simulink library "EMD"  (R2021b)
settings: Solver=VariableStepAuto  StartTime=0.0  StopTime=10.0  RelTol=1e-3
libraries: $bdroot x2
settings Model: Creator=Szalay  LastModifiedBy=Szalay

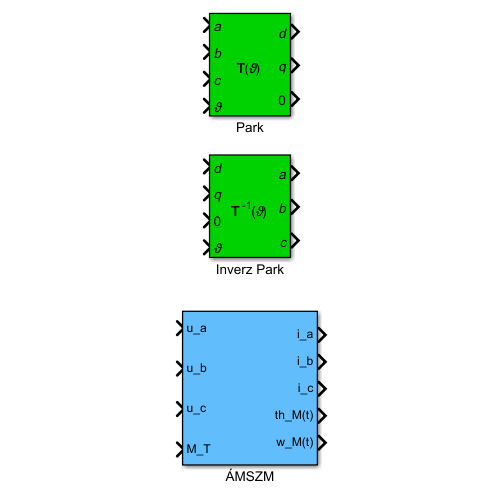
[thumbnail: Simulink's stored preview of the top-level diagram]
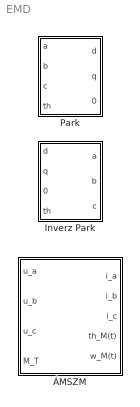
== system EMD ==
  Inverz Park : Subsystem
      mask Display:
      | % Bemenetek
      | port_label('input', 1, '\itd', 'texmode', 'on');
      | port_label('input', 2, '\itq', 'texmode', 'on');
      | port_label('input', 3, '0', 'texmode', 'on');
      | 
      | port_label('input', 4, '\it\vartheta', 'texmode', 'on');
      | 
      | % Kimenetek
      | port_label('output', 1, '\ita', 'texmode', 'on');
      | port_label('output', 2, '\itb', 'texmode', 'on');
      | port_label('output', 3, '\itc', 'texmode', 'on');
      | 
      | % Felirat
      | text( ...
      | 	0.5, 0.5, '{\bfT}^{ -1}({\it\vartheta})', ...
      | 	'texmode', 'on', ...
      | 	'HorizontalAlignment', 'center' ...
      | 	);
  Park : Subsystem
      mask Display:
      | % Bemenetek
      | port_label('input', 1, '\ita', 'texmode', 'on');
      | port_label('input', 2, '\itb', 'texmode', 'on');
      | port_label('input', 3, '\itc', 'texmode', 'on');
      | 
      | port_label('input', 4, '\it\vartheta', 'texmode', 'on');
      | 
      | % Kimenetek
      | port_label('output', 1, '\itd', 'texmode', 'on');
      | port_label('output', 2, '\itq', 'texmode', 'on');
      | port_label('output', 3, '0', 'texmode', 'on');
      | 
      | % Felirat
      | text( ...
      | 	0.5, 0.5, '{\bfT}({\it\vartheta})', ...
      | 	'texmode', 'on', ...
      | 	'HorizontalAlignment', 'center' ...
      | 	);
  ÁMSZM : Subsystem

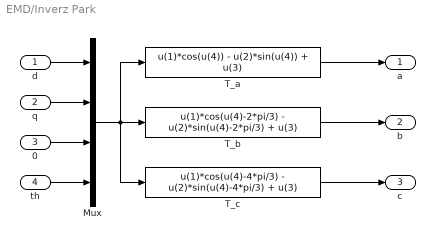
== system EMD/Inverz Park ==
  d : Inport
  q : Inport  Port=2
  0 : Inport  Port=3
  th : Inport  Port=4
  Mux : Mux
  T_a : MATLABFcn  MATLABFcn=u(1)*cos(u(4)) - u(2)*sin(u(4)) + u(3)
  T_b : MATLABFcn  MATLABFcn=u(1)*cos(u(4)-2*pi/3) - u(2)*sin(u(4)-2*pi/3) + u(3)
  T_c : MATLABFcn  MATLABFcn=u(1)*cos(u(4)-4*pi/3) - u(2)*sin(u(4)-4*pi/3) + u(3)
  a : Outport
  b : Outport  Port=2
  c : Outport  Port=3
  wires:
  0/1 -> Mux/3
  d/1 -> Mux/1
  th/1 -> Mux/4
  T_c/1 -> c/1
  q/1 -> Mux/2
  T_b/1 -> b/1
  T_a/1 -> a/1
  Mux/1 -> T_b/1, T_c/1, T_a/1

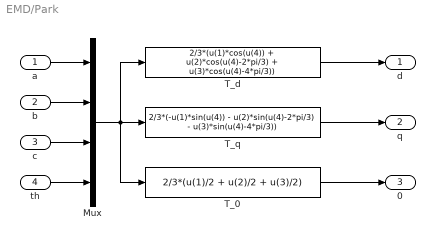
== system EMD/Park ==
  a : Inport
  b : Inport  Port=2
  c : Inport  Port=3
  th : Inport  Port=4
  Mux : Mux
  T_0 : MATLABFcn  MATLABFcn=2/3*(u(1)/2 + u(2)/2 + u(3)/2)
  T_d : MATLABFcn  MATLABFcn=2/3*(u(1)*cos(u(4)) + u(2)*cos(u(4)-2*pi/3) + u(3)*cos(u(4)-4*pi/3))
  T_q : MATLABFcn  MATLABFcn=2/3*(-u(1)*sin(u(4)) - u(2)*sin(u(4)-2*pi/3) - u(3)*sin(u(4)-4*pi/3))
  d : Outport
  q : Outport  Port=2
  0 : Outport  Port=3
  wires:
  Mux/1 -> T_d/1, T_0/1, T_q/1
  T_d/1 -> d/1
  T_q/1 -> q/1
  b/1 -> Mux/2
  T_0/1 -> 0/1
  th/1 -> Mux/4
  a/1 -> Mux/1
  c/1 -> Mux/3

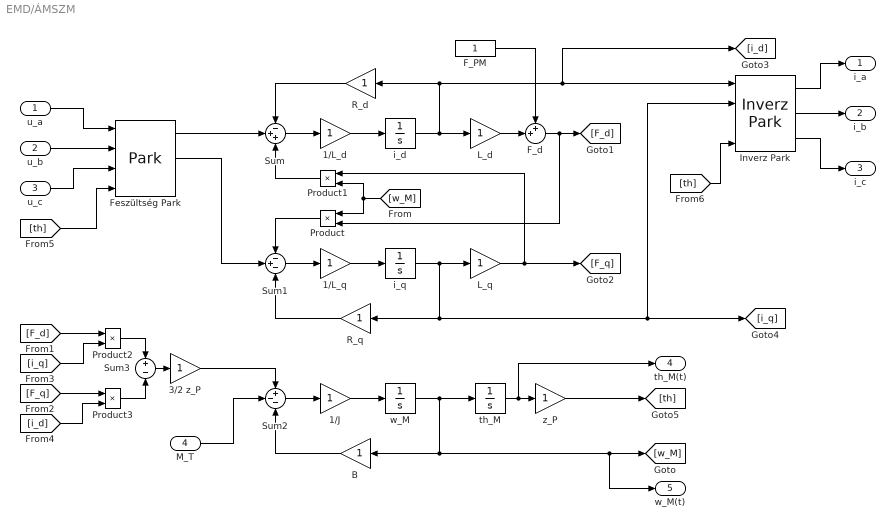
== system EMD/ÁMSZM ==
  u_a : Inport
  u_b : Inport  Port=2
  u_c : Inport  Port=3
  M_T : Inport  Port=4
  1/J : Gain
  1/L_d : Gain
  1/L_q : Gain
  3/2 z_P : Gain
  B : Gain
  F_PM : Constant
  F_d : Sum  Inputs=++|
  Feszültség Park : $bdroot/Park  SystemSampleTime=-1  VariantActivationTime=update diagram  Latency=0  AutoFrameSizeCalculation=off
  Inverz Park : $bdroot/Inverz Park  SystemSampleTime=-1  VariantActivationTime=update diagram  Latency=0  AutoFrameSizeCalculation=off
  L_d : Gain
  L_q : Gain
  Product{,1..3} (4 alike) : Product
  R_d : Gain
  R_q : Gain
  Sum : Sum  Inputs=-++
  Sum1 : Sum  Inputs=-+-
  Sum2 : Sum  Inputs=+--
  Sum3 : Sum  Inputs=+|-
  i_d : Integrator
  i_q : Integrator
  th_M : Integrator
  w_M : Integrator
  z_P : Gain
  i_a : Outport
  i_b : Outport  Port=2
  i_c : Outport  Port=3
  th_M(t) : Outport  Port=4
  w_M(t) : Outport  Port=5
  wires:
  Sum/1 -> 1/L_d/1
  [w_M] -> Product/1, Product1/2
  F_d/1 -> [F_d], Product/2
  Inverz Park/1 -> i_a/1
  R_q/1 -> Sum1/3
  3/2 z_P/1 -> Sum2/1
  Sum1/1 -> 1/L_q/1
  w_M/1 -> th_M/1, w_M(t)/1, [w_M], B/1
  Inverz Park/3 -> i_c/1
  z_P/1 -> [th]
  1/L_q/1 -> i_q/1
  Product/1 -> Sum1/1
  Product3/1 -> Sum3/2
  u_b/1 -> Feszültség Park/2
  Product1/1 -> Sum/3
  L_q/1 -> [F_q], Product1/1
  Sum3/1 -> 3/2 z_P/1
  i_d/1 -> R_d/1, Inverz Park/1, [i_d], L_d/1
  i_q/1 -> L_q/1, [i_q], Inverz Park/2, R_q/1
  1/L_d/1 -> i_d/1
  L_d/1 -> F_d/2
  Sum2/1 -> 1/J/1
  [i_d] -> Product3/2
  Product2/1 -> Sum3/1
  [F_q] -> Product3/1
  R_d/1 -> Sum/1
  F_PM/1 -> F_d/1
  1/J/1 -> w_M/1
  [F_d] -> Product2/1
  B/1 -> Sum2/3
  Feszültség Park/1 -> Sum/2
  Feszültség Park/2 -> Sum1/2
  u_a/1 -> Feszültség Park/1
  [th] -> Feszültség Park/4
  [i_q] -> Product2/2
  M_T/1 -> Sum2/2
  th_M/1 -> th_M(t)/1, z_P/1
  u_c/1 -> Feszültség Park/3
  Inverz Park/2 -> i_b/1
  [th] -> Inverz Park/4
